simulink model "gm_ZynqBF_2tx_fpga"  (R2018b)
settings: Solver=FixedStepDiscrete  StartTime=0.0  StopTime=10.0  FixedStep=(1/420e3)/128  RelTol=1e-3
undefined symbols (not defined in the file or in its folder): a, b, c
libraries: hdlsllib x873, simulink x349
(part 37 of 40)

== system gm_ZynqBF_2tx_fpga/channel_estimator/peakdetect_ch2/correlator2/sum_elements_q_instance4 ==
  din : Inport  OutDataTypeStr=fixdt(1, 32, 16)  PortDimensions=[8]  SampleTime=1.86011904761905e-08
  start : Inport  Port=2  OutDataTypeStr=boolean  PortDimensions=1  SampleTime=1.86011904761905e-08
  Add : Sum  AccumDataTypeStr=fixdt(1, 33, 16)  OutDataTypeStr=fixdt(1, 32, 16)  SampleTime=1.86011904761905e-08
  Compare To Constant1 : simulink/Logic and Bit Operations/Compare To Constant  relop===  const=fi(0,0,3,0,'hex','7')  OutDataTypeStr=boolean
  Compare To Constant2 : simulink/Logic and Bit Operations/Compare To Constant  relop===  const=fi(0,0,1,0,'hex','1')  OutDataTypeStr=boolean
  Constant : Constant  Value=0  OutDataTypeStr=fixdt(1, 32, 16)  SampleTime=-1
  Constant1 : Constant  Value=0  OutDataTypeStr=fixdt(1, 16, 15)  SampleTime=-1
  Data Type Conversion : DataTypeConversion  OutDataTypeStr=uint8  SampleTime=1.86011904761905e-08
  Delay1 : Delay  DelayLength=double(1)  InitialCondition=0  InputProcessing=Inherited  SampleTime=1.86011904761905e-08
  HDL Counter : hdlsllib/Sources/HDL Counter  CountType=Free running  CountInit=double(0)  CountStep=double(1)  CountMax=25  CountFromType=Initial value  CountFrom=double(0)  CountResetPort=on  CountLoadPort=off  CountEnbPort=on  CountDirPort=off  CountDataType=Unsigned  CountWordLen=3  CountFracLen=0  CountSampTime=1.86011904761905e-08
      settings: SourceProductBaseCode=HD
  HDL Counter1 : hdlsllib/Sources/HDL Counter  CountType=Free running  CountInit=double(0)  CountStep=double(1)  CountMax=25  CountFromType=Initial value  CountFrom=double(0)  CountResetPort=off  CountLoadPort=off  CountEnbPort=on  CountDirPort=off  CountDataType=Unsigned  CountWordLen=1  CountFracLen=0  CountSampTime=1.86011904761905e-08
      settings: SourceProductBaseCode=HD
  Logical Operator : Logic  Operator=OR  AllPortsSameDT=off  OutDataTypeStr=boolean  SampleTime=1.86011904761905e-08
  Selector : Selector  IndexMode=Zero-based  SampleTime=1.86011904761905e-08  IndexOptions=Starting index (port)  Indices=double([1 3])  OutputSizes=double(1)
  Switch : Switch  Criteria=u2 ~= 0  Threshold=double(0)  OutDataTypeStr=fixdt(1, 32, 16)  SampleTime=1.86011904761905e-08
  Switch1 : Switch  Criteria=u2 ~= 0  Threshold=double(0)  OutDataTypeStr=fixdt(1, 32, 16)  SampleTime=1.86011904761905e-08
  dout : Outport
  vout : Outport  Port=2
  wires:
  Switch/1 -> Add/2
  Delay1/1 -> Switch/3
  HDL Counter1/1 -> Compare To Constant2/1
  Logical Operator/1 -> HDL Counter1/1
  start/1 -> Switch/2, HDL Counter/1, Logical Operator/1
  din/1 -> Selector/1
  Add/1 -> Delay1/1, dout/1
  Compare To Constant1/1 -> Logical Operator/2, vout/1
  Compare To Constant2/1 -> HDL Counter/2, Switch1/2
  Constant/1 -> Switch/1
  Constant1/1 -> Switch1/3
  Data Type Conversion/1 -> Selector/2
  HDL Counter/1 -> Compare To Constant1/1, Data Type Conversion/1
  Selector/1 -> Switch1/1
  Switch1/1 -> Add/1

== system gm_ZynqBF_2tx_fpga/channel_estimator/peakdetect_ch2/correlator2/sum_elements_q_instance5 ==
  din : Inport  OutDataTypeStr=fixdt(1, 32, 16)  PortDimensions=[8]  SampleTime=1.86011904761905e-08
  start : Inport  Port=2  OutDataTypeStr=boolean  PortDimensions=1  SampleTime=1.86011904761905e-08
  Add : Sum  AccumDataTypeStr=fixdt(1, 33, 16)  OutDataTypeStr=fixdt(1, 32, 16)  SampleTime=1.86011904761905e-08
  Compare To Constant1 : simulink/Logic and Bit Operations/Compare To Constant  relop===  const=fi(0,0,3,0,'hex','7')  OutDataTypeStr=boolean
  Compare To Constant2 : simulink/Logic and Bit Operations/Compare To Constant  relop===  const=fi(0,0,1,0,'hex','1')  OutDataTypeStr=boolean
  Constant : Constant  Value=0  OutDataTypeStr=fixdt(1, 32, 16)  SampleTime=-1
  Constant1 : Constant  Value=0  OutDataTypeStr=fixdt(1, 16, 15)  SampleTime=-1
  Data Type Conversion : DataTypeConversion  OutDataTypeStr=uint8  SampleTime=1.86011904761905e-08
  Delay1 : Delay  DelayLength=double(1)  InitialCondition=0  InputProcessing=Inherited  SampleTime=1.86011904761905e-08
  HDL Counter : hdlsllib/Sources/HDL Counter  CountType=Free running  CountInit=double(0)  CountStep=double(1)  CountMax=25  CountFromType=Initial value  CountFrom=double(0)  CountResetPort=on  CountLoadPort=off  CountEnbPort=on  CountDirPort=off  CountDataType=Unsigned  CountWordLen=3  CountFracLen=0  CountSampTime=1.86011904761905e-08
      settings: SourceProductBaseCode=HD
  HDL Counter1 : hdlsllib/Sources/HDL Counter  CountType=Free running  CountInit=double(0)  CountStep=double(1)  CountMax=25  CountFromType=Initial value  CountFrom=double(0)  CountResetPort=off  CountLoadPort=off  CountEnbPort=on  CountDirPort=off  CountDataType=Unsigned  CountWordLen=1  CountFracLen=0  CountSampTime=1.86011904761905e-08
      settings: SourceProductBaseCode=HD
  Logical Operator : Logic  Operator=OR  AllPortsSameDT=off  OutDataTypeStr=boolean  SampleTime=1.86011904761905e-08
  Selector : Selector  IndexMode=Zero-based  SampleTime=1.86011904761905e-08  IndexOptions=Starting index (port)  Indices=double([1 3])  OutputSizes=double(1)
  Switch : Switch  Criteria=u2 ~= 0  Threshold=double(0)  OutDataTypeStr=fixdt(1, 32, 16)  SampleTime=1.86011904761905e-08
  Switch1 : Switch  Criteria=u2 ~= 0  Threshold=double(0)  OutDataTypeStr=fixdt(1, 32, 16)  SampleTime=1.86011904761905e-08
  dout : Outport
  vout : Outport  Port=2
  wires:
  Switch/1 -> Add/2
  Delay1/1 -> Switch/3
  HDL Counter1/1 -> Compare To Constant2/1
  Logical Operator/1 -> HDL Counter1/1
  start/1 -> Switch/2, HDL Counter/1, Logical Operator/1
  din/1 -> Selector/1
  Add/1 -> Delay1/1, dout/1
  Compare To Constant1/1 -> Logical Operator/2, vout/1
  Compare To Constant2/1 -> HDL Counter/2, Switch1/2
  Constant/1 -> Switch/1
  Constant1/1 -> Switch1/3
  Data Type Conversion/1 -> Selector/2
  HDL Counter/1 -> Compare To Constant1/1, Data Type Conversion/1
  Selector/1 -> Switch1/1
  Switch1/1 -> Add/1

== system gm_ZynqBF_2tx_fpga/channel_estimator/peakdetect_ch2/correlator2/sum_elements_q_instance6 ==
  din : Inport  OutDataTypeStr=fixdt(1, 32, 16)  PortDimensions=[8]  SampleTime=1.86011904761905e-08
  start : Inport  Port=2  OutDataTypeStr=boolean  PortDimensions=1  SampleTime=1.86011904761905e-08
  Add : Sum  AccumDataTypeStr=fixdt(1, 33, 16)  OutDataTypeStr=fixdt(1, 32, 16)  SampleTime=1.86011904761905e-08
  Compare To Constant1 : simulink/Logic and Bit Operations/Compare To Constant  relop===  const=fi(0,0,3,0,'hex','7')  OutDataTypeStr=boolean
  Compare To Constant2 : simulink/Logic and Bit Operations/Compare To Constant  relop===  const=fi(0,0,1,0,'hex','1')  OutDataTypeStr=boolean
  Constant : Constant  Value=0  OutDataTypeStr=fixdt(1, 32, 16)  SampleTime=-1
  Constant1 : Constant  Value=0  OutDataTypeStr=fixdt(1, 16, 15)  SampleTime=-1
  Data Type Conversion : DataTypeConversion  OutDataTypeStr=uint8  SampleTime=1.86011904761905e-08
  Delay1 : Delay  DelayLength=double(1)  InitialCondition=0  InputProcessing=Inherited  SampleTime=1.86011904761905e-08
  HDL Counter : hdlsllib/Sources/HDL Counter  CountType=Free running  CountInit=double(0)  CountStep=double(1)  CountMax=25  CountFromType=Initial value  CountFrom=double(0)  CountResetPort=on  CountLoadPort=off  CountEnbPort=on  CountDirPort=off  CountDataType=Unsigned  CountWordLen=3  CountFracLen=0  CountSampTime=1.86011904761905e-08
      settings: SourceProductBaseCode=HD
  HDL Counter1 : hdlsllib/Sources/HDL Counter  CountType=Free running  CountInit=double(0)  CountStep=double(1)  CountMax=25  CountFromType=Initial value  CountFrom=double(0)  CountResetPort=off  CountLoadPort=off  CountEnbPort=on  CountDirPort=off  CountDataType=Unsigned  CountWordLen=1  CountFracLen=0  CountSampTime=1.86011904761905e-08
      settings: SourceProductBaseCode=HD
  Logical Operator : Logic  Operator=OR  AllPortsSameDT=off  OutDataTypeStr=boolean  SampleTime=1.86011904761905e-08
  Selector : Selector  IndexMode=Zero-based  SampleTime=1.86011904761905e-08  IndexOptions=Starting index (port)  Indices=double([1 3])  OutputSizes=double(1)
  Switch : Switch  Criteria=u2 ~= 0  Threshold=double(0)  OutDataTypeStr=fixdt(1, 32, 16)  SampleTime=1.86011904761905e-08
  Switch1 : Switch  Criteria=u2 ~= 0  Threshold=double(0)  OutDataTypeStr=fixdt(1, 32, 16)  SampleTime=1.86011904761905e-08
  dout : Outport
  vout : Outport  Port=2
  wires:
  Switch/1 -> Add/2
  Delay1/1 -> Switch/3
  HDL Counter1/1 -> Compare To Constant2/1
  Logical Operator/1 -> HDL Counter1/1
  start/1 -> Switch/2, HDL Counter/1, Logical Operator/1
  din/1 -> Selector/1
  Add/1 -> Delay1/1, dout/1
  Compare To Constant1/1 -> Logical Operator/2, vout/1
  Compare To Constant2/1 -> HDL Counter/2, Switch1/2
  Constant/1 -> Switch/1
  Constant1/1 -> Switch1/3
  Data Type Conversion/1 -> Selector/2
  HDL Counter/1 -> Compare To Constant1/1, Data Type Conversion/1
  Selector/1 -> Switch1/1
  Switch1/1 -> Add/1

== system gm_ZynqBF_2tx_fpga/channel_estimator/peakdetect_ch2/correlator2/sum_elements_q_instance7 ==
  din : Inport  OutDataTypeStr=fixdt(1, 32, 16)  PortDimensions=[8]  SampleTime=1.86011904761905e-08
  start : Inport  Port=2  OutDataTypeStr=boolean  PortDimensions=1  SampleTime=1.86011904761905e-08
  Add : Sum  AccumDataTypeStr=fixdt(1, 33, 16)  OutDataTypeStr=fixdt(1, 32, 16)  SampleTime=1.86011904761905e-08
  Compare To Constant1 : simulink/Logic and Bit Operations/Compare To Constant  relop===  const=fi(0,0,3,0,'hex','7')  OutDataTypeStr=boolean
  Compare To Constant2 : simulink/Logic and Bit Operations/Compare To Constant  relop===  const=fi(0,0,1,0,'hex','1')  OutDataTypeStr=boolean
  Constant : Constant  Value=0  OutDataTypeStr=fixdt(1, 32, 16)  SampleTime=-1
  Constant1 : Constant  Value=0  OutDataTypeStr=fixdt(1, 16, 15)  SampleTime=-1
  Data Type Conversion : DataTypeConversion  OutDataTypeStr=uint8  SampleTime=1.86011904761905e-08
  Delay1 : Delay  DelayLength=double(1)  InitialCondition=0  InputProcessing=Inherited  SampleTime=1.86011904761905e-08
  HDL Counter : hdlsllib/Sources/HDL Counter  CountType=Free running  CountInit=double(0)  CountStep=double(1)  CountMax=25  CountFromType=Initial value  CountFrom=double(0)  CountResetPort=on  CountLoadPort=off  CountEnbPort=on  CountDirPort=off  CountDataType=Unsigned  CountWordLen=3  CountFracLen=0  CountSampTime=1.86011904761905e-08
      settings: SourceProductBaseCode=HD
  HDL Counter1 : hdlsllib/Sources/HDL Counter  CountType=Free running  CountInit=double(0)  CountStep=double(1)  CountMax=25  CountFromType=Initial value  CountFrom=double(0)  CountResetPort=off  CountLoadPort=off  CountEnbPort=on  CountDirPort=off  CountDataType=Unsigned  CountWordLen=1  CountFracLen=0  CountSampTime=1.86011904761905e-08
      settings: SourceProductBaseCode=HD
  Logical Operator : Logic  Operator=OR  AllPortsSameDT=off  OutDataTypeStr=boolean  SampleTime=1.86011904761905e-08
  Selector : Selector  IndexMode=Zero-based  SampleTime=1.86011904761905e-08  IndexOptions=Starting index (port)  Indices=double([1 3])  OutputSizes=double(1)
  Switch : Switch  Criteria=u2 ~= 0  Threshold=double(0)  OutDataTypeStr=fixdt(1, 32, 16)  SampleTime=1.86011904761905e-08
  Switch1 : Switch  Criteria=u2 ~= 0  Threshold=double(0)  OutDataTypeStr=fixdt(1, 32, 16)  SampleTime=1.86011904761905e-08
  dout : Outport
  vout : Outport  Port=2
  wires:
  Switch/1 -> Add/2
  Delay1/1 -> Switch/3
  HDL Counter1/1 -> Compare To Constant2/1
  Logical Operator/1 -> HDL Counter1/1
  start/1 -> Switch/2, HDL Counter/1, Logical Operator/1
  din/1 -> Selector/1
  Add/1 -> Delay1/1, dout/1
  Compare To Constant1/1 -> Logical Operator/2, vout/1
  Compare To Constant2/1 -> HDL Counter/2, Switch1/2
  Constant/1 -> Switch/1
  Constant1/1 -> Switch1/3
  Data Type Conversion/1 -> Selector/2
  HDL Counter/1 -> Compare To Constant1/1, Data Type Conversion/1
  Selector/1 -> Switch1/1
  Switch1/1 -> Add/1

== system gm_ZynqBF_2tx_fpga/channel_estimator/peakdetect_ch2/correlator2/sum_elements_q_instance8 ==
  din : Inport  OutDataTypeStr=fixdt(1, 32, 16)  PortDimensions=[8]  SampleTime=1.86011904761905e-08
  start : Inport  Port=2  OutDataTypeStr=boolean  PortDimensions=1  SampleTime=1.86011904761905e-08
  Add : Sum  AccumDataTypeStr=fixdt(1, 33, 16)  OutDataTypeStr=fixdt(1, 32, 16)  SampleTime=1.86011904761905e-08
  Compare To Constant1 : simulink/Logic and Bit Operations/Compare To Constant  relop===  const=fi(0,0,3,0,'hex','7')  OutDataTypeStr=boolean
  Compare To Constant2 : simulink/Logic and Bit Operations/Compare To Constant  relop===  const=fi(0,0,1,0,'hex','1')  OutDataTypeStr=boolean
  Constant : Constant  Value=0  OutDataTypeStr=fixdt(1, 32, 16)  SampleTime=-1
  Constant1 : Constant  Value=0  OutDataTypeStr=fixdt(1, 16, 15)  SampleTime=-1
  Data Type Conversion : DataTypeConversion  OutDataTypeStr=uint8  SampleTime=1.86011904761905e-08
  Delay1 : Delay  DelayLength=double(1)  InitialCondition=0  InputProcessing=Inherited  SampleTime=1.86011904761905e-08
  HDL Counter : hdlsllib/Sources/HDL Counter  CountType=Free running  CountInit=double(0)  CountStep=double(1)  CountMax=25  CountFromType=Initial value  CountFrom=double(0)  CountResetPort=on  CountLoadPort=off  CountEnbPort=on  CountDirPort=off  CountDataType=Unsigned  CountWordLen=3  CountFracLen=0  CountSampTime=1.86011904761905e-08
      settings: SourceProductBaseCode=HD
  HDL Counter1 : hdlsllib/Sources/HDL Counter  CountType=Free running  CountInit=double(0)  CountStep=double(1)  CountMax=25  CountFromType=Initial value  CountFrom=double(0)  CountResetPort=off  CountLoadPort=off  CountEnbPort=on  CountDirPort=off  CountDataType=Unsigned  CountWordLen=1  CountFracLen=0  CountSampTime=1.86011904761905e-08
      settings: SourceProductBaseCode=HD
  Logical Operator : Logic  Operator=OR  AllPortsSameDT=off  OutDataTypeStr=boolean  SampleTime=1.86011904761905e-08
  Selector : Selector  IndexMode=Zero-based  SampleTime=1.86011904761905e-08  IndexOptions=Starting index (port)  Indices=double([1 3])  OutputSizes=double(1)
  Switch : Switch  Criteria=u2 ~= 0  Threshold=double(0)  OutDataTypeStr=fixdt(1, 32, 16)  SampleTime=1.86011904761905e-08
  Switch1 : Switch  Criteria=u2 ~= 0  Threshold=double(0)  OutDataTypeStr=fixdt(1, 32, 16)  SampleTime=1.86011904761905e-08
  dout : Outport
  vout : Outport  Port=2
  wires:
  Switch/1 -> Add/2
  Delay1/1 -> Switch/3
  HDL Counter1/1 -> Compare To Constant2/1
  Logical Operator/1 -> HDL Counter1/1
  start/1 -> Switch/2, HDL Counter/1, Logical Operator/1
  din/1 -> Selector/1
  Add/1 -> Delay1/1, dout/1
  Compare To Constant1/1 -> Logical Operator/2, vout/1
  Compare To Constant2/1 -> HDL Counter/2, Switch1/2
  Constant/1 -> Switch/1
  Constant1/1 -> Switch1/3
  Data Type Conversion/1 -> Selector/2
  HDL Counter/1 -> Compare To Constant1/1, Data Type Conversion/1
  Selector/1 -> Switch1/1
  Switch1/1 -> Add/1

== system gm_ZynqBF_2tx_fpga/channel_estimator/peakdetect_ch1/correlator1/rx_ram_i_instance1/get_bit ==
  u : Inport  OutDataTypeStr=fixdt(0, 64, 0)  PortDimensions=1  SampleTime=1.86011904761905e-08
  ind : Inport  Port=2  OutDataTypeStr=fixdt(0, 9, 0)  PortDimensions=1  SampleTime=1.86011904761905e-08
  get_bit : MATLAB Function  TreatAsAtomicUnit=on
  y : Outport
  wires:
  u/1 -> get_bit/1(u)
  ind/1 -> get_bit/2(ind)
  get_bit/1(y) -> y/1

== system gm_ZynqBF_2tx_fpga/channel_estimator/peakdetect_ch1/correlator1/rx_ram_i_instance10/get_bit ==
  u : Inport  OutDataTypeStr=fixdt(0, 64, 0)  PortDimensions=1  SampleTime=1.86011904761905e-08
  ind : Inport  Port=2  OutDataTypeStr=fixdt(0, 9, 0)  PortDimensions=1  SampleTime=1.86011904761905e-08
  get_bit : MATLAB Function  TreatAsAtomicUnit=on
  y : Outport
  wires:
  get_bit/1(y) -> y/1
  ind/1 -> get_bit/2(ind)
  u/1 -> get_bit/1(u)

== system gm_ZynqBF_2tx_fpga/channel_estimator/peakdetect_ch1/correlator1/rx_ram_i_instance11/get_bit ==
  u : Inport  OutDataTypeStr=fixdt(0, 64, 0)  PortDimensions=1  SampleTime=1.86011904761905e-08
  ind : Inport  Port=2  OutDataTypeStr=fixdt(0, 9, 0)  PortDimensions=1  SampleTime=1.86011904761905e-08
  get_bit : MATLAB Function  TreatAsAtomicUnit=on
  y : Outport
  wires:
  get_bit/1(y) -> y/1
  ind/1 -> get_bit/2(ind)
  u/1 -> get_bit/1(u)

== system gm_ZynqBF_2tx_fpga/channel_estimator/peakdetect_ch1/correlator1/rx_ram_i_instance12/get_bit ==
  u : Inport  OutDataTypeStr=fixdt(0, 64, 0)  PortDimensions=1  SampleTime=1.86011904761905e-08
  ind : Inport  Port=2  OutDataTypeStr=fixdt(0, 9, 0)  PortDimensions=1  SampleTime=1.86011904761905e-08
  get_bit : MATLAB Function  TreatAsAtomicUnit=on
  y : Outport
  wires:
  get_bit/1(y) -> y/1
  ind/1 -> get_bit/2(ind)
  u/1 -> get_bit/1(u)

== system gm_ZynqBF_2tx_fpga/channel_estimator/peakdetect_ch1/correlator1/rx_ram_i_instance13/get_bit ==
  u : Inport  OutDataTypeStr=fixdt(0, 64, 0)  PortDimensions=1  SampleTime=1.86011904761905e-08
  ind : Inport  Port=2  OutDataTypeStr=fixdt(0, 9, 0)  PortDimensions=1  SampleTime=1.86011904761905e-08
  get_bit : MATLAB Function  TreatAsAtomicUnit=on
  y : Outport
  wires:
  get_bit/1(y) -> y/1
  ind/1 -> get_bit/2(ind)
  u/1 -> get_bit/1(u)

== system gm_ZynqBF_2tx_fpga/channel_estimator/peakdetect_ch1/correlator1/rx_ram_i_instance14/get_bit ==
  u : Inport  OutDataTypeStr=fixdt(0, 64, 0)  PortDimensions=1  SampleTime=1.86011904761905e-08
  ind : Inport  Port=2  OutDataTypeStr=fixdt(0, 9, 0)  PortDimensions=1  SampleTime=1.86011904761905e-08
  get_bit : MATLAB Function  TreatAsAtomicUnit=on
  y : Outport
  wires:
  get_bit/1(y) -> y/1
  ind/1 -> get_bit/2(ind)
  u/1 -> get_bit/1(u)

== system gm_ZynqBF_2tx_fpga/channel_estimator/peakdetect_ch1/correlator1/rx_ram_i_instance15/get_bit ==
  u : Inport  OutDataTypeStr=fixdt(0, 64, 0)  PortDimensions=1  SampleTime=1.86011904761905e-08
  ind : Inport  Port=2  OutDataTypeStr=fixdt(0, 9, 0)  PortDimensions=1  SampleTime=1.86011904761905e-08
  get_bit : MATLAB Function  TreatAsAtomicUnit=on
  y : Outport
  wires:
  get_bit/1(y) -> y/1
  ind/1 -> get_bit/2(ind)
  u/1 -> get_bit/1(u)

== system gm_ZynqBF_2tx_fpga/channel_estimator/peakdetect_ch1/correlator1/rx_ram_i_instance16/get_bit ==
  u : Inport  OutDataTypeStr=fixdt(0, 64, 0)  PortDimensions=1  SampleTime=1.86011904761905e-08
  ind : Inport  Port=2  OutDataTypeStr=fixdt(0, 9, 0)  PortDimensions=1  SampleTime=1.86011904761905e-08
  get_bit : MATLAB Function  TreatAsAtomicUnit=on
  y : Outport
  wires:
  get_bit/1(y) -> y/1
  ind/1 -> get_bit/2(ind)
  u/1 -> get_bit/1(u)

== system gm_ZynqBF_2tx_fpga/channel_estimator/peakdetect_ch1/correlator1/rx_ram_i_instance17/get_bit ==
  u : Inport  OutDataTypeStr=fixdt(0, 64, 0)  PortDimensions=1  SampleTime=1.86011904761905e-08
  ind : Inport  Port=2  OutDataTypeStr=fixdt(0, 9, 0)  PortDimensions=1  SampleTime=1.86011904761905e-08
  get_bit : MATLAB Function  TreatAsAtomicUnit=on
  y : Outport
  wires:
  get_bit/1(y) -> y/1
  ind/1 -> get_bit/2(ind)
  u/1 -> get_bit/1(u)

== system gm_ZynqBF_2tx_fpga/channel_estimator/peakdetect_ch1/correlator1/rx_ram_i_instance18/get_bit ==
  u : Inport  OutDataTypeStr=fixdt(0, 64, 0)  PortDimensions=1  SampleTime=1.86011904761905e-08
  ind : Inport  Port=2  OutDataTypeStr=fixdt(0, 9, 0)  PortDimensions=1  SampleTime=1.86011904761905e-08
  get_bit : MATLAB Function  TreatAsAtomicUnit=on
  y : Outport
  wires:
  get_bit/1(y) -> y/1
  ind/1 -> get_bit/2(ind)
  u/1 -> get_bit/1(u)

== system gm_ZynqBF_2tx_fpga/channel_estimator/peakdetect_ch1/correlator1/rx_ram_i_instance19/get_bit ==
  u : Inport  OutDataTypeStr=fixdt(0, 64, 0)  PortDimensions=1  SampleTime=1.86011904761905e-08
  ind : Inport  Port=2  OutDataTypeStr=fixdt(0, 9, 0)  PortDimensions=1  SampleTime=1.86011904761905e-08
  get_bit : MATLAB Function  TreatAsAtomicUnit=on
  y : Outport
  wires:
  get_bit/1(y) -> y/1
  ind/1 -> get_bit/2(ind)
  u/1 -> get_bit/1(u)

== system gm_ZynqBF_2tx_fpga/channel_estimator/peakdetect_ch1/correlator1/rx_ram_i_instance2/get_bit ==
  u : Inport  OutDataTypeStr=fixdt(0, 64, 0)  PortDimensions=1  SampleTime=1.86011904761905e-08
  ind : Inport  Port=2  OutDataTypeStr=fixdt(0, 9, 0)  PortDimensions=1  SampleTime=1.86011904761905e-08
  get_bit : MATLAB Function  TreatAsAtomicUnit=on
  y : Outport
  wires:
  get_bit/1(y) -> y/1
  ind/1 -> get_bit/2(ind)
  u/1 -> get_bit/1(u)

== system gm_ZynqBF_2tx_fpga/channel_estimator/peakdetect_ch1/correlator1/rx_ram_i_instance20/get_bit ==
  u : Inport  OutDataTypeStr=fixdt(0, 64, 0)  PortDimensions=1  SampleTime=1.86011904761905e-08
  ind : Inport  Port=2  OutDataTypeStr=fixdt(0, 9, 0)  PortDimensions=1  SampleTime=1.86011904761905e-08
  get_bit : MATLAB Function  TreatAsAtomicUnit=on
  y : Outport
  wires:
  get_bit/1(y) -> y/1
  ind/1 -> get_bit/2(ind)
  u/1 -> get_bit/1(u)

== system gm_ZynqBF_2tx_fpga/channel_estimator/peakdetect_ch1/correlator1/rx_ram_i_instance21/get_bit ==
  u : Inport  OutDataTypeStr=fixdt(0, 64, 0)  PortDimensions=1  SampleTime=1.86011904761905e-08
  ind : Inport  Port=2  OutDataTypeStr=fixdt(0, 9, 0)  PortDimensions=1  SampleTime=1.86011904761905e-08
  get_bit : MATLAB Function  TreatAsAtomicUnit=on
  y : Outport
  wires:
  get_bit/1(y) -> y/1
  ind/1 -> get_bit/2(ind)
  u/1 -> get_bit/1(u)

== system gm_ZynqBF_2tx_fpga/channel_estimator/peakdetect_ch1/correlator1/rx_ram_i_instance22/get_bit ==
  u : Inport  OutDataTypeStr=fixdt(0, 64, 0)  PortDimensions=1  SampleTime=1.86011904761905e-08
  ind : Inport  Port=2  OutDataTypeStr=fixdt(0, 9, 0)  PortDimensions=1  SampleTime=1.86011904761905e-08
  get_bit : MATLAB Function  TreatAsAtomicUnit=on
  y : Outport
  wires:
  get_bit/1(y) -> y/1
  ind/1 -> get_bit/2(ind)
  u/1 -> get_bit/1(u)

== system gm_ZynqBF_2tx_fpga/channel_estimator/peakdetect_ch1/correlator1/rx_ram_i_instance23/get_bit ==
  u : Inport  OutDataTypeStr=fixdt(0, 64, 0)  PortDimensions=1  SampleTime=1.86011904761905e-08
  ind : Inport  Port=2  OutDataTypeStr=fixdt(0, 9, 0)  PortDimensions=1  SampleTime=1.86011904761905e-08
  get_bit : MATLAB Function  TreatAsAtomicUnit=on
  y : Outport
  wires:
  get_bit/1(y) -> y/1
  ind/1 -> get_bit/2(ind)
  u/1 -> get_bit/1(u)

== system gm_ZynqBF_2tx_fpga/channel_estimator/peakdetect_ch1/correlator1/rx_ram_i_instance24/get_bit ==
  u : Inport  OutDataTypeStr=fixdt(0, 64, 0)  PortDimensions=1  SampleTime=1.86011904761905e-08
  ind : Inport  Port=2  OutDataTypeStr=fixdt(0, 9, 0)  PortDimensions=1  SampleTime=1.86011904761905e-08
  get_bit : MATLAB Function  TreatAsAtomicUnit=on
  y : Outport
  wires:
  get_bit/1(y) -> y/1
  ind/1 -> get_bit/2(ind)
  u/1 -> get_bit/1(u)

== system gm_ZynqBF_2tx_fpga/channel_estimator/peakdetect_ch1/correlator1/rx_ram_i_instance25/get_bit ==
  u : Inport  OutDataTypeStr=fixdt(0, 64, 0)  PortDimensions=1  SampleTime=1.86011904761905e-08
  ind : Inport  Port=2  OutDataTypeStr=fixdt(0, 9, 0)  PortDimensions=1  SampleTime=1.86011904761905e-08
  get_bit : MATLAB Function  TreatAsAtomicUnit=on
  y : Outport
  wires:
  get_bit/1(y) -> y/1
  ind/1 -> get_bit/2(ind)
  u/1 -> get_bit/1(u)

== system gm_ZynqBF_2tx_fpga/channel_estimator/peakdetect_ch1/correlator1/rx_ram_i_instance26/get_bit ==
  u : Inport  OutDataTypeStr=fixdt(0, 64, 0)  PortDimensions=1  SampleTime=1.86011904761905e-08
  ind : Inport  Port=2  OutDataTypeStr=fixdt(0, 9, 0)  PortDimensions=1  SampleTime=1.86011904761905e-08
  get_bit : MATLAB Function  TreatAsAtomicUnit=on
  y : Outport
  wires:
  get_bit/1(y) -> y/1
  ind/1 -> get_bit/2(ind)
  u/1 -> get_bit/1(u)

== system gm_ZynqBF_2tx_fpga/channel_estimator/peakdetect_ch1/correlator1/rx_ram_i_instance27/get_bit ==
  u : Inport  OutDataTypeStr=fixdt(0, 64, 0)  PortDimensions=1  SampleTime=1.86011904761905e-08
  ind : Inport  Port=2  OutDataTypeStr=fixdt(0, 9, 0)  PortDimensions=1  SampleTime=1.86011904761905e-08
  get_bit : MATLAB Function  TreatAsAtomicUnit=on
  y : Outport
  wires:
  get_bit/1(y) -> y/1
  ind/1 -> get_bit/2(ind)
  u/1 -> get_bit/1(u)

== system gm_ZynqBF_2tx_fpga/channel_estimator/peakdetect_ch1/correlator1/rx_ram_i_instance28/get_bit ==
  u : Inport  OutDataTypeStr=fixdt(0, 64, 0)  PortDimensions=1  SampleTime=1.86011904761905e-08
  ind : Inport  Port=2  OutDataTypeStr=fixdt(0, 9, 0)  PortDimensions=1  SampleTime=1.86011904761905e-08
  get_bit : MATLAB Function  TreatAsAtomicUnit=on
  y : Outport
  wires:
  get_bit/1(y) -> y/1
  ind/1 -> get_bit/2(ind)
  u/1 -> get_bit/1(u)

== system gm_ZynqBF_2tx_fpga/channel_estimator/peakdetect_ch1/correlator1/rx_ram_i_instance29/get_bit ==
  u : Inport  OutDataTypeStr=fixdt(0, 64, 0)  PortDimensions=1  SampleTime=1.86011904761905e-08
  ind : Inport  Port=2  OutDataTypeStr=fixdt(0, 9, 0)  PortDimensions=1  SampleTime=1.86011904761905e-08
  get_bit : MATLAB Function  TreatAsAtomicUnit=on
  y : Outport
  wires:
  get_bit/1(y) -> y/1
  ind/1 -> get_bit/2(ind)
  u/1 -> get_bit/1(u)

== system gm_ZynqBF_2tx_fpga/channel_estimator/peakdetect_ch1/correlator1/rx_ram_i_instance3/get_bit ==
  u : Inport  OutDataTypeStr=fixdt(0, 64, 0)  PortDimensions=1  SampleTime=1.86011904761905e-08
  ind : Inport  Port=2  OutDataTypeStr=fixdt(0, 9, 0)  PortDimensions=1  SampleTime=1.86011904761905e-08
  get_bit : MATLAB Function  TreatAsAtomicUnit=on
  y : Outport
  wires:
  get_bit/1(y) -> y/1
  ind/1 -> get_bit/2(ind)
  u/1 -> get_bit/1(u)

== system gm_ZynqBF_2tx_fpga/channel_estimator/peakdetect_ch1/correlator1/rx_ram_i_instance30/get_bit ==
  u : Inport  OutDataTypeStr=fixdt(0, 64, 0)  PortDimensions=1  SampleTime=1.86011904761905e-08
  ind : Inport  Port=2  OutDataTypeStr=fixdt(0, 9, 0)  PortDimensions=1  SampleTime=1.86011904761905e-08
  get_bit : MATLAB Function  TreatAsAtomicUnit=on
  y : Outport
  wires:
  get_bit/1(y) -> y/1
  ind/1 -> get_bit/2(ind)
  u/1 -> get_bit/1(u)

== system gm_ZynqBF_2tx_fpga/channel_estimator/peakdetect_ch1/correlator1/rx_ram_i_instance31/get_bit ==
  u : Inport  OutDataTypeStr=fixdt(0, 64, 0)  PortDimensions=1  SampleTime=1.86011904761905e-08
  ind : Inport  Port=2  OutDataTypeStr=fixdt(0, 9, 0)  PortDimensions=1  SampleTime=1.86011904761905e-08
  get_bit : MATLAB Function  TreatAsAtomicUnit=on
  y : Outport
  wires:
  get_bit/1(y) -> y/1
  ind/1 -> get_bit/2(ind)
  u/1 -> get_bit/1(u)

== system gm_ZynqBF_2tx_fpga/channel_estimator/peakdetect_ch1/correlator1/rx_ram_i_instance32/get_bit ==
  u : Inport  OutDataTypeStr=fixdt(0, 64, 0)  PortDimensions=1  SampleTime=1.86011904761905e-08
  ind : Inport  Port=2  OutDataTypeStr=fixdt(0, 9, 0)  PortDimensions=1  SampleTime=1.86011904761905e-08
  get_bit : MATLAB Function  TreatAsAtomicUnit=on
  y : Outport
  wires:
  get_bit/1(y) -> y/1
  ind/1 -> get_bit/2(ind)
  u/1 -> get_bit/1(u)

== system gm_ZynqBF_2tx_fpga/channel_estimator/peakdetect_ch1/correlator1/rx_ram_i_instance33/get_bit ==
  u : Inport  OutDataTypeStr=fixdt(0, 64, 0)  PortDimensions=1  SampleTime=1.86011904761905e-08
  ind : Inport  Port=2  OutDataTypeStr=fixdt(0, 9, 0)  PortDimensions=1  SampleTime=1.86011904761905e-08
  get_bit : MATLAB Function  TreatAsAtomicUnit=on
  y : Outport
  wires:
  get_bit/1(y) -> y/1
  ind/1 -> get_bit/2(ind)
  u/1 -> get_bit/1(u)

== system gm_ZynqBF_2tx_fpga/channel_estimator/peakdetect_ch1/correlator1/rx_ram_i_instance34/get_bit ==
  u : Inport  OutDataTypeStr=fixdt(0, 64, 0)  PortDimensions=1  SampleTime=1.86011904761905e-08
  ind : Inport  Port=2  OutDataTypeStr=fixdt(0, 9, 0)  PortDimensions=1  SampleTime=1.86011904761905e-08
  get_bit : MATLAB Function  TreatAsAtomicUnit=on
  y : Outport
  wires:
  get_bit/1(y) -> y/1
  ind/1 -> get_bit/2(ind)
  u/1 -> get_bit/1(u)

== system gm_ZynqBF_2tx_fpga/channel_estimator/peakdetect_ch1/correlator1/rx_ram_i_instance35/get_bit ==
  u : Inport  OutDataTypeStr=fixdt(0, 64, 0)  PortDimensions=1  SampleTime=1.86011904761905e-08
  ind : Inport  Port=2  OutDataTypeStr=fixdt(0, 9, 0)  PortDimensions=1  SampleTime=1.86011904761905e-08
  get_bit : MATLAB Function  TreatAsAtomicUnit=on
  y : Outport
  wires:
  get_bit/1(y) -> y/1
  ind/1 -> get_bit/2(ind)
  u/1 -> get_bit/1(u)

== system gm_ZynqBF_2tx_fpga/channel_estimator/peakdetect_ch1/correlator1/rx_ram_i_instance36/get_bit ==
  u : Inport  OutDataTypeStr=fixdt(0, 64, 0)  PortDimensions=1  SampleTime=1.86011904761905e-08
  ind : Inport  Port=2  OutDataTypeStr=fixdt(0, 9, 0)  PortDimensions=1  SampleTime=1.86011904761905e-08
  get_bit : MATLAB Function  TreatAsAtomicUnit=on
  y : Outport
  wires:
  get_bit/1(y) -> y/1
  ind/1 -> get_bit/2(ind)
  u/1 -> get_bit/1(u)

== system gm_ZynqBF_2tx_fpga/channel_estimator/peakdetect_ch1/correlator1/rx_ram_i_instance37/get_bit ==
  u : Inport  OutDataTypeStr=fixdt(0, 64, 0)  PortDimensions=1  SampleTime=1.86011904761905e-08
  ind : Inport  Port=2  OutDataTypeStr=fixdt(0, 9, 0)  PortDimensions=1  SampleTime=1.86011904761905e-08
  get_bit : MATLAB Function  TreatAsAtomicUnit=on
  y : Outport
  wires:
  get_bit/1(y) -> y/1
  ind/1 -> get_bit/2(ind)
  u/1 -> get_bit/1(u)

== system gm_ZynqBF_2tx_fpga/channel_estimator/peakdetect_ch1/correlator1/rx_ram_i_instance38/get_bit ==
  u : Inport  OutDataTypeStr=fixdt(0, 64, 0)  PortDimensions=1  SampleTime=1.86011904761905e-08
  ind : Inport  Port=2  OutDataTypeStr=fixdt(0, 9, 0)  PortDimensions=1  SampleTime=1.86011904761905e-08
  get_bit : MATLAB Function  TreatAsAtomicUnit=on
  y : Outport
  wires:
  get_bit/1(y) -> y/1
  ind/1 -> get_bit/2(ind)
  u/1 -> get_bit/1(u)

== system gm_ZynqBF_2tx_fpga/channel_estimator/peakdetect_ch1/correlator1/rx_ram_i_instance39/get_bit ==
  u : Inport  OutDataTypeStr=fixdt(0, 64, 0)  PortDimensions=1  SampleTime=1.86011904761905e-08
  ind : Inport  Port=2  OutDataTypeStr=fixdt(0, 9, 0)  PortDimensions=1  SampleTime=1.86011904761905e-08
  get_bit : MATLAB Function  TreatAsAtomicUnit=on
  y : Outport
  wires:
  get_bit/1(y) -> y/1
  ind/1 -> get_bit/2(ind)
  u/1 -> get_bit/1(u)

== system gm_ZynqBF_2tx_fpga/channel_estimator/peakdetect_ch1/correlator1/rx_ram_i_instance4/get_bit ==
  u : Inport  OutDataTypeStr=fixdt(0, 64, 0)  PortDimensions=1  SampleTime=1.86011904761905e-08
  ind : Inport  Port=2  OutDataTypeStr=fixdt(0, 9, 0)  PortDimensions=1  SampleTime=1.86011904761905e-08
  get_bit : MATLAB Function  TreatAsAtomicUnit=on
  y : Outport
  wires:
  get_bit/1(y) -> y/1
  ind/1 -> get_bit/2(ind)
  u/1 -> get_bit/1(u)

== system gm_ZynqBF_2tx_fpga/channel_estimator/peakdetect_ch1/correlator1/rx_ram_i_instance40/get_bit ==
  u : Inport  OutDataTypeStr=fixdt(0, 64, 0)  PortDimensions=1  SampleTime=1.86011904761905e-08
  ind : Inport  Port=2  OutDataTypeStr=fixdt(0, 9, 0)  PortDimensions=1  SampleTime=1.86011904761905e-08
  get_bit : MATLAB Function  TreatAsAtomicUnit=on
  y : Outport
  wires:
  get_bit/1(y) -> y/1
  ind/1 -> get_bit/2(ind)
  u/1 -> get_bit/1(u)

== system gm_ZynqBF_2tx_fpga/channel_estimator/peakdetect_ch1/correlator1/rx_ram_i_instance41/get_bit ==
  u : Inport  OutDataTypeStr=fixdt(0, 64, 0)  PortDimensions=1  SampleTime=1.86011904761905e-08
  ind : Inport  Port=2  OutDataTypeStr=fixdt(0, 9, 0)  PortDimensions=1  SampleTime=1.86011904761905e-08
  get_bit : MATLAB Function  TreatAsAtomicUnit=on
  y : Outport
  wires:
  get_bit/1(y) -> y/1
  ind/1 -> get_bit/2(ind)
  u/1 -> get_bit/1(u)

== system gm_ZynqBF_2tx_fpga/channel_estimator/peakdetect_ch1/correlator1/rx_ram_i_instance42/get_bit ==
  u : Inport  OutDataTypeStr=fixdt(0, 64, 0)  PortDimensions=1  SampleTime=1.86011904761905e-08
  ind : Inport  Port=2  OutDataTypeStr=fixdt(0, 9, 0)  PortDimensions=1  SampleTime=1.86011904761905e-08
  get_bit : MATLAB Function  TreatAsAtomicUnit=on
  y : Outport
  wires:
  get_bit/1(y) -> y/1
  ind/1 -> get_bit/2(ind)
  u/1 -> get_bit/1(u)

== system gm_ZynqBF_2tx_fpga/channel_estimator/peakdetect_ch1/correlator1/rx_ram_i_instance43/get_bit ==
  u : Inport  OutDataTypeStr=fixdt(0, 64, 0)  PortDimensions=1  SampleTime=1.86011904761905e-08
  ind : Inport  Port=2  OutDataTypeStr=fixdt(0, 9, 0)  PortDimensions=1  SampleTime=1.86011904761905e-08
  get_bit : MATLAB Function  TreatAsAtomicUnit=on
  y : Outport
  wires:
  get_bit/1(y) -> y/1
  ind/1 -> get_bit/2(ind)
  u/1 -> get_bit/1(u)

== system gm_ZynqBF_2tx_fpga/channel_estimator/peakdetect_ch1/correlator1/rx_ram_i_instance44/get_bit ==
  u : Inport  OutDataTypeStr=fixdt(0, 64, 0)  PortDimensions=1  SampleTime=1.86011904761905e-08
  ind : Inport  Port=2  OutDataTypeStr=fixdt(0, 9, 0)  PortDimensions=1  SampleTime=1.86011904761905e-08
  get_bit : MATLAB Function  TreatAsAtomicUnit=on
  y : Outport
  wires:
  get_bit/1(y) -> y/1
  ind/1 -> get_bit/2(ind)
  u/1 -> get_bit/1(u)

== system gm_ZynqBF_2tx_fpga/channel_estimator/peakdetect_ch1/correlator1/rx_ram_i_instance45/get_bit ==
  u : Inport  OutDataTypeStr=fixdt(0, 64, 0)  PortDimensions=1  SampleTime=1.86011904761905e-08
  ind : Inport  Port=2  OutDataTypeStr=fixdt(0, 9, 0)  PortDimensions=1  SampleTime=1.86011904761905e-08
  get_bit : MATLAB Function  TreatAsAtomicUnit=on
  y : Outport
  wires:
  get_bit/1(y) -> y/1
  ind/1 -> get_bit/2(ind)
  u/1 -> get_bit/1(u)

== system gm_ZynqBF_2tx_fpga/channel_estimator/peakdetect_ch1/correlator1/rx_ram_i_instance46/get_bit ==
  u : Inport  OutDataTypeStr=fixdt(0, 64, 0)  PortDimensions=1  SampleTime=1.86011904761905e-08
  ind : Inport  Port=2  OutDataTypeStr=fixdt(0, 9, 0)  PortDimensions=1  SampleTime=1.86011904761905e-08
  get_bit : MATLAB Function  TreatAsAtomicUnit=on
  y : Outport
  wires:
  get_bit/1(y) -> y/1
  ind/1 -> get_bit/2(ind)
  u/1 -> get_bit/1(u)

== system gm_ZynqBF_2tx_fpga/channel_estimator/peakdetect_ch1/correlator1/rx_ram_i_instance47/get_bit ==
  u : Inport  OutDataTypeStr=fixdt(0, 64, 0)  PortDimensions=1  SampleTime=1.86011904761905e-08
  ind : Inport  Port=2  OutDataTypeStr=fixdt(0, 9, 0)  PortDimensions=1  SampleTime=1.86011904761905e-08
  get_bit : MATLAB Function  TreatAsAtomicUnit=on
  y : Outport
  wires:
  get_bit/1(y) -> y/1
  ind/1 -> get_bit/2(ind)
  u/1 -> get_bit/1(u)

== system gm_ZynqBF_2tx_fpga/channel_estimator/peakdetect_ch1/correlator1/rx_ram_i_instance48/get_bit ==
  u : Inport  OutDataTypeStr=fixdt(0, 64, 0)  PortDimensions=1  SampleTime=1.86011904761905e-08
  ind : Inport  Port=2  OutDataTypeStr=fixdt(0, 9, 0)  PortDimensions=1  SampleTime=1.86011904761905e-08
  get_bit : MATLAB Function  TreatAsAtomicUnit=on
  y : Outport
  wires:
  get_bit/1(y) -> y/1
  ind/1 -> get_bit/2(ind)
  u/1 -> get_bit/1(u)

== system gm_ZynqBF_2tx_fpga/channel_estimator/peakdetect_ch1/correlator1/rx_ram_i_instance49/get_bit ==
  u : Inport  OutDataTypeStr=fixdt(0, 64, 0)  PortDimensions=1  SampleTime=1.86011904761905e-08
  ind : Inport  Port=2  OutDataTypeStr=fixdt(0, 9, 0)  PortDimensions=1  SampleTime=1.86011904761905e-08
  get_bit : MATLAB Function  TreatAsAtomicUnit=on
  y : Outport
  wires:
  get_bit/1(y) -> y/1
  ind/1 -> get_bit/2(ind)
  u/1 -> get_bit/1(u)

== system gm_ZynqBF_2tx_fpga/channel_estimator/peakdetect_ch1/correlator1/rx_ram_i_instance5/get_bit ==
  u : Inport  OutDataTypeStr=fixdt(0, 64, 0)  PortDimensions=1  SampleTime=1.86011904761905e-08
  ind : Inport  Port=2  OutDataTypeStr=fixdt(0, 9, 0)  PortDimensions=1  SampleTime=1.86011904761905e-08
  get_bit : MATLAB Function  TreatAsAtomicUnit=on
  y : Outport
  wires:
  get_bit/1(y) -> y/1
  ind/1 -> get_bit/2(ind)
  u/1 -> get_bit/1(u)

== system gm_ZynqBF_2tx_fpga/channel_estimator/peakdetect_ch1/correlator1/rx_ram_i_instance50/get_bit ==
  u : Inport  OutDataTypeStr=fixdt(0, 64, 0)  PortDimensions=1  SampleTime=1.86011904761905e-08
  ind : Inport  Port=2  OutDataTypeStr=fixdt(0, 9, 0)  PortDimensions=1  SampleTime=1.86011904761905e-08
  get_bit : MATLAB Function  TreatAsAtomicUnit=on
  y : Outport
  wires:
  get_bit/1(y) -> y/1
  ind/1 -> get_bit/2(ind)
  u/1 -> get_bit/1(u)

== system gm_ZynqBF_2tx_fpga/channel_estimator/peakdetect_ch1/correlator1/rx_ram_i_instance51/get_bit ==
  u : Inport  OutDataTypeStr=fixdt(0, 64, 0)  PortDimensions=1  SampleTime=1.86011904761905e-08
  ind : Inport  Port=2  OutDataTypeStr=fixdt(0, 9, 0)  PortDimensions=1  SampleTime=1.86011904761905e-08
  get_bit : MATLAB Function  TreatAsAtomicUnit=on
  y : Outport
  wires:
  get_bit/1(y) -> y/1
  ind/1 -> get_bit/2(ind)
  u/1 -> get_bit/1(u)

== system gm_ZynqBF_2tx_fpga/channel_estimator/peakdetect_ch1/correlator1/rx_ram_i_instance52/get_bit ==
  u : Inport  OutDataTypeStr=fixdt(0, 64, 0)  PortDimensions=1  SampleTime=1.86011904761905e-08
  ind : Inport  Port=2  OutDataTypeStr=fixdt(0, 9, 0)  PortDimensions=1  SampleTime=1.86011904761905e-08
  get_bit : MATLAB Function  TreatAsAtomicUnit=on
  y : Outport
  wires:
  get_bit/1(y) -> y/1
  ind/1 -> get_bit/2(ind)
  u/1 -> get_bit/1(u)

== system gm_ZynqBF_2tx_fpga/channel_estimator/peakdetect_ch1/correlator1/rx_ram_i_instance53/get_bit ==
  u : Inport  OutDataTypeStr=fixdt(0, 64, 0)  PortDimensions=1  SampleTime=1.86011904761905e-08
  ind : Inport  Port=2  OutDataTypeStr=fixdt(0, 9, 0)  PortDimensions=1  SampleTime=1.86011904761905e-08
  get_bit : MATLAB Function  TreatAsAtomicUnit=on
  y : Outport
  wires:
  get_bit/1(y) -> y/1
  ind/1 -> get_bit/2(ind)
  u/1 -> get_bit/1(u)

== system gm_ZynqBF_2tx_fpga/channel_estimator/peakdetect_ch1/correlator1/rx_ram_i_instance54/get_bit ==
  u : Inport  OutDataTypeStr=fixdt(0, 64, 0)  PortDimensions=1  SampleTime=1.86011904761905e-08
  ind : Inport  Port=2  OutDataTypeStr=fixdt(0, 9, 0)  PortDimensions=1  SampleTime=1.86011904761905e-08
  get_bit : MATLAB Function  TreatAsAtomicUnit=on
  y : Outport
  wires:
  get_bit/1(y) -> y/1
  ind/1 -> get_bit/2(ind)
  u/1 -> get_bit/1(u)

== system gm_ZynqBF_2tx_fpga/channel_estimator/peakdetect_ch1/correlator1/rx_ram_i_instance55/get_bit ==
  u : Inport  OutDataTypeStr=fixdt(0, 64, 0)  PortDimensions=1  SampleTime=1.86011904761905e-08
  ind : Inport  Port=2  OutDataTypeStr=fixdt(0, 9, 0)  PortDimensions=1  SampleTime=1.86011904761905e-08
  get_bit : MATLAB Function  TreatAsAtomicUnit=on
  y : Outport
  wires:
  get_bit/1(y) -> y/1
  ind/1 -> get_bit/2(ind)
  u/1 -> get_bit/1(u)

== system gm_ZynqBF_2tx_fpga/channel_estimator/peakdetect_ch1/correlator1/rx_ram_i_instance56/get_bit ==
  u : Inport  OutDataTypeStr=fixdt(0, 64, 0)  PortDimensions=1  SampleTime=1.86011904761905e-08
  ind : Inport  Port=2  OutDataTypeStr=fixdt(0, 9, 0)  PortDimensions=1  SampleTime=1.86011904761905e-08
  get_bit : MATLAB Function  TreatAsAtomicUnit=on
  y : Outport
  wires:
  get_bit/1(y) -> y/1
  ind/1 -> get_bit/2(ind)
  u/1 -> get_bit/1(u)

== system gm_ZynqBF_2tx_fpga/channel_estimator/peakdetect_ch1/correlator1/rx_ram_i_instance57/get_bit ==
  u : Inport  OutDataTypeStr=fixdt(0, 64, 0)  PortDimensions=1  SampleTime=1.86011904761905e-08
  ind : Inport  Port=2  OutDataTypeStr=fixdt(0, 9, 0)  PortDimensions=1  SampleTime=1.86011904761905e-08
  get_bit : MATLAB Function  TreatAsAtomicUnit=on
  y : Outport
  wires:
  get_bit/1(y) -> y/1
  ind/1 -> get_bit/2(ind)
  u/1 -> get_bit/1(u)

== system gm_ZynqBF_2tx_fpga/channel_estimator/peakdetect_ch1/correlator1/rx_ram_i_instance58/get_bit ==
  u : Inport  OutDataTypeStr=fixdt(0, 64, 0)  PortDimensions=1  SampleTime=1.86011904761905e-08
  ind : Inport  Port=2  OutDataTypeStr=fixdt(0, 9, 0)  PortDimensions=1  SampleTime=1.86011904761905e-08
  get_bit : MATLAB Function  TreatAsAtomicUnit=on
  y : Outport
  wires:
  get_bit/1(y) -> y/1
  ind/1 -> get_bit/2(ind)
  u/1 -> get_bit/1(u)

== system gm_ZynqBF_2tx_fpga/channel_estimator/peakdetect_ch1/correlator1/rx_ram_i_instance59/get_bit ==
  u : Inport  OutDataTypeStr=fixdt(0, 64, 0)  PortDimensions=1  SampleTime=1.86011904761905e-08
  ind : Inport  Port=2  OutDataTypeStr=fixdt(0, 9, 0)  PortDimensions=1  SampleTime=1.86011904761905e-08
  get_bit : MATLAB Function  TreatAsAtomicUnit=on
  y : Outport
  wires:
  get_bit/1(y) -> y/1
  ind/1 -> get_bit/2(ind)
  u/1 -> get_bit/1(u)

== system gm_ZynqBF_2tx_fpga/channel_estimator/peakdetect_ch1/correlator1/rx_ram_i_instance6/get_bit ==
  u : Inport  OutDataTypeStr=fixdt(0, 64, 0)  PortDimensions=1  SampleTime=1.86011904761905e-08
  ind : Inport  Port=2  OutDataTypeStr=fixdt(0, 9, 0)  PortDimensions=1  SampleTime=1.86011904761905e-08
  get_bit : MATLAB Function  TreatAsAtomicUnit=on
  y : Outport
  wires:
  get_bit/1(y) -> y/1
  ind/1 -> get_bit/2(ind)
  u/1 -> get_bit/1(u)

== system gm_ZynqBF_2tx_fpga/channel_estimator/peakdetect_ch1/correlator1/rx_ram_i_instance60/get_bit ==
  u : Inport  OutDataTypeStr=fixdt(0, 64, 0)  PortDimensions=1  SampleTime=1.86011904761905e-08
  ind : Inport  Port=2  OutDataTypeStr=fixdt(0, 9, 0)  PortDimensions=1  SampleTime=1.86011904761905e-08
  get_bit : MATLAB Function  TreatAsAtomicUnit=on
  y : Outport
  wires:
  get_bit/1(y) -> y/1
  ind/1 -> get_bit/2(ind)
  u/1 -> get_bit/1(u)

== system gm_ZynqBF_2tx_fpga/channel_estimator/peakdetect_ch1/correlator1/rx_ram_i_instance61/get_bit ==
  u : Inport  OutDataTypeStr=fixdt(0, 64, 0)  PortDimensions=1  SampleTime=1.86011904761905e-08
  ind : Inport  Port=2  OutDataTypeStr=fixdt(0, 9, 0)  PortDimensions=1  SampleTime=1.86011904761905e-08
  get_bit : MATLAB Function  TreatAsAtomicUnit=on
  y : Outport
  wires:
  get_bit/1(y) -> y/1
  ind/1 -> get_bit/2(ind)
  u/1 -> get_bit/1(u)

== system gm_ZynqBF_2tx_fpga/channel_estimator/peakdetect_ch1/correlator1/rx_ram_i_instance62/get_bit ==
  u : Inport  OutDataTypeStr=fixdt(0, 64, 0)  PortDimensions=1  SampleTime=1.86011904761905e-08
  ind : Inport  Port=2  OutDataTypeStr=fixdt(0, 9, 0)  PortDimensions=1  SampleTime=1.86011904761905e-08
  get_bit : MATLAB Function  TreatAsAtomicUnit=on
  y : Outport
  wires:
  get_bit/1(y) -> y/1
  ind/1 -> get_bit/2(ind)
  u/1 -> get_bit/1(u)

== system gm_ZynqBF_2tx_fpga/channel_estimator/peakdetect_ch1/correlator1/rx_ram_i_instance63/get_bit ==
  u : Inport  OutDataTypeStr=fixdt(0, 64, 0)  PortDimensions=1  SampleTime=1.86011904761905e-08
  ind : Inport  Port=2  OutDataTypeStr=fixdt(0, 9, 0)  PortDimensions=1  SampleTime=1.86011904761905e-08
  get_bit : MATLAB Function  TreatAsAtomicUnit=on
  y : Outport
  wires:
  get_bit/1(y) -> y/1
  ind/1 -> get_bit/2(ind)
  u/1 -> get_bit/1(u)

== system gm_ZynqBF_2tx_fpga/channel_estimator/peakdetect_ch1/correlator1/rx_ram_i_instance64/get_bit ==
  u : Inport  OutDataTypeStr=fixdt(0, 64, 0)  PortDimensions=1  SampleTime=1.86011904761905e-08
  ind : Inport  Port=2  OutDataTypeStr=fixdt(0, 9, 0)  PortDimensions=1  SampleTime=1.86011904761905e-08
  get_bit : MATLAB Function  TreatAsAtomicUnit=on
  y : Outport
  wires:
  get_bit/1(y) -> y/1
  ind/1 -> get_bit/2(ind)
  u/1 -> get_bit/1(u)

== system gm_ZynqBF_2tx_fpga/channel_estimator/peakdetect_ch1/correlator1/rx_ram_i_instance7/get_bit ==
  u : Inport  OutDataTypeStr=fixdt(0, 64, 0)  PortDimensions=1  SampleTime=1.86011904761905e-08
  ind : Inport  Port=2  OutDataTypeStr=fixdt(0, 9, 0)  PortDimensions=1  SampleTime=1.86011904761905e-08
  get_bit : MATLAB Function  TreatAsAtomicUnit=on
  y : Outport
  wires:
  get_bit/1(y) -> y/1
  ind/1 -> get_bit/2(ind)
  u/1 -> get_bit/1(u)

== system gm_ZynqBF_2tx_fpga/channel_estimator/peakdetect_ch1/correlator1/rx_ram_i_instance8/get_bit ==
  u : Inport  OutDataTypeStr=fixdt(0, 64, 0)  PortDimensions=1  SampleTime=1.86011904761905e-08
  ind : Inport  Port=2  OutDataTypeStr=fixdt(0, 9, 0)  PortDimensions=1  SampleTime=1.86011904761905e-08
  get_bit : MATLAB Function  TreatAsAtomicUnit=on
  y : Outport
  wires:
  get_bit/1(y) -> y/1
  ind/1 -> get_bit/2(ind)
  u/1 -> get_bit/1(u)

== system gm_ZynqBF_2tx_fpga/channel_estimator/peakdetect_ch1/correlator1/rx_ram_i_instance9/get_bit ==
  u : Inport  OutDataTypeStr=fixdt(0, 64, 0)  PortDimensions=1  SampleTime=1.86011904761905e-08
  ind : Inport  Port=2  OutDataTypeStr=fixdt(0, 9, 0)  PortDimensions=1  SampleTime=1.86011904761905e-08
  get_bit : MATLAB Function  TreatAsAtomicUnit=on
  y : Outport
  wires:
  get_bit/1(y) -> y/1
  ind/1 -> get_bit/2(ind)
  u/1 -> get_bit/1(u)

== system gm_ZynqBF_2tx_fpga/channel_estimator/peakdetect_ch1/correlator1/rx_ram_q_instance1/get_bit ==
  u : Inport  OutDataTypeStr=fixdt(0, 64, 0)  PortDimensions=1  SampleTime=1.86011904761905e-08
  ind : Inport  Port=2  OutDataTypeStr=fixdt(0, 9, 0)  PortDimensions=1  SampleTime=1.86011904761905e-08
  get_bit : MATLAB Function  TreatAsAtomicUnit=on
  y : Outport
  wires:
  get_bit/1(y) -> y/1
  ind/1 -> get_bit/2(ind)
  u/1 -> get_bit/1(u)

== system gm_ZynqBF_2tx_fpga/channel_estimator/peakdetect_ch1/correlator1/rx_ram_q_instance10/get_bit ==
  u : Inport  OutDataTypeStr=fixdt(0, 64, 0)  PortDimensions=1  SampleTime=1.86011904761905e-08
  ind : Inport  Port=2  OutDataTypeStr=fixdt(0, 9, 0)  PortDimensions=1  SampleTime=1.86011904761905e-08
  get_bit : MATLAB Function  TreatAsAtomicUnit=on
  y : Outport
  wires:
  get_bit/1(y) -> y/1
  ind/1 -> get_bit/2(ind)
  u/1 -> get_bit/1(u)

== system gm_ZynqBF_2tx_fpga/channel_estimator/peakdetect_ch1/correlator1/rx_ram_q_instance11/get_bit ==
  u : Inport  OutDataTypeStr=fixdt(0, 64, 0)  PortDimensions=1  SampleTime=1.86011904761905e-08
  ind : Inport  Port=2  OutDataTypeStr=fixdt(0, 9, 0)  PortDimensions=1  SampleTime=1.86011904761905e-08
  get_bit : MATLAB Function  TreatAsAtomicUnit=on
  y : Outport
  wires:
  get_bit/1(y) -> y/1
  ind/1 -> get_bit/2(ind)
  u/1 -> get_bit/1(u)

== system gm_ZynqBF_2tx_fpga/channel_estimator/peakdetect_ch1/correlator1/rx_ram_q_instance12/get_bit ==
  u : Inport  OutDataTypeStr=fixdt(0, 64, 0)  PortDimensions=1  SampleTime=1.86011904761905e-08
  ind : Inport  Port=2  OutDataTypeStr=fixdt(0, 9, 0)  PortDimensions=1  SampleTime=1.86011904761905e-08
  get_bit : MATLAB Function  TreatAsAtomicUnit=on
  y : Outport
  wires:
  get_bit/1(y) -> y/1
  ind/1 -> get_bit/2(ind)
  u/1 -> get_bit/1(u)

== system gm_ZynqBF_2tx_fpga/channel_estimator/peakdetect_ch1/correlator1/rx_ram_q_instance13/get_bit ==
  u : Inport  OutDataTypeStr=fixdt(0, 64, 0)  PortDimensions=1  SampleTime=1.86011904761905e-08
  ind : Inport  Port=2  OutDataTypeStr=fixdt(0, 9, 0)  PortDimensions=1  SampleTime=1.86011904761905e-08
  get_bit : MATLAB Function  TreatAsAtomicUnit=on
  y : Outport
  wires:
  get_bit/1(y) -> y/1
  ind/1 -> get_bit/2(ind)
  u/1 -> get_bit/1(u)

== system gm_ZynqBF_2tx_fpga/channel_estimator/peakdetect_ch1/correlator1/rx_ram_q_instance14/get_bit ==
  u : Inport  OutDataTypeStr=fixdt(0, 64, 0)  PortDimensions=1  SampleTime=1.86011904761905e-08
  ind : Inport  Port=2  OutDataTypeStr=fixdt(0, 9, 0)  PortDimensions=1  SampleTime=1.86011904761905e-08
  get_bit : MATLAB Function  TreatAsAtomicUnit=on
  y : Outport
  wires:
  get_bit/1(y) -> y/1
  ind/1 -> get_bit/2(ind)
  u/1 -> get_bit/1(u)

== system gm_ZynqBF_2tx_fpga/channel_estimator/peakdetect_ch1/correlator1/rx_ram_q_instance15/get_bit ==
  u : Inport  OutDataTypeStr=fixdt(0, 64, 0)  PortDimensions=1  SampleTime=1.86011904761905e-08
  ind : Inport  Port=2  OutDataTypeStr=fixdt(0, 9, 0)  PortDimensions=1  SampleTime=1.86011904761905e-08
  get_bit : MATLAB Function  TreatAsAtomicUnit=on
  y : Outport
  wires:
  get_bit/1(y) -> y/1
  ind/1 -> get_bit/2(ind)
  u/1 -> get_bit/1(u)

== system gm_ZynqBF_2tx_fpga/channel_estimator/peakdetect_ch1/correlator1/rx_ram_q_instance16/get_bit ==
  u : Inport  OutDataTypeStr=fixdt(0, 64, 0)  PortDimensions=1  SampleTime=1.86011904761905e-08
  ind : Inport  Port=2  OutDataTypeStr=fixdt(0, 9, 0)  PortDimensions=1  SampleTime=1.86011904761905e-08
  get_bit : MATLAB Function  TreatAsAtomicUnit=on
  y : Outport
  wires:
  get_bit/1(y) -> y/1
  ind/1 -> get_bit/2(ind)
  u/1 -> get_bit/1(u)

== system gm_ZynqBF_2tx_fpga/channel_estimator/peakdetect_ch1/correlator1/rx_ram_q_instance17/get_bit ==
  u : Inport  OutDataTypeStr=fixdt(0, 64, 0)  PortDimensions=1  SampleTime=1.86011904761905e-08
  ind : Inport  Port=2  OutDataTypeStr=fixdt(0, 9, 0)  PortDimensions=1  SampleTime=1.86011904761905e-08
  get_bit : MATLAB Function  TreatAsAtomicUnit=on
  y : Outport
  wires:
  get_bit/1(y) -> y/1
  ind/1 -> get_bit/2(ind)
  u/1 -> get_bit/1(u)

== system gm_ZynqBF_2tx_fpga/channel_estimator/peakdetect_ch1/correlator1/rx_ram_q_instance18/get_bit ==
  u : Inport  OutDataTypeStr=fixdt(0, 64, 0)  PortDimensions=1  SampleTime=1.86011904761905e-08
  ind : Inport  Port=2  OutDataTypeStr=fixdt(0, 9, 0)  PortDimensions=1  SampleTime=1.86011904761905e-08
  get_bit : MATLAB Function  TreatAsAtomicUnit=on
  y : Outport
  wires:
  get_bit/1(y) -> y/1
  ind/1 -> get_bit/2(ind)
  u/1 -> get_bit/1(u)

== system gm_ZynqBF_2tx_fpga/channel_estimator/peakdetect_ch1/correlator1/rx_ram_q_instance19/get_bit ==
  u : Inport  OutDataTypeStr=fixdt(0, 64, 0)  PortDimensions=1  SampleTime=1.86011904761905e-08
  ind : Inport  Port=2  OutDataTypeStr=fixdt(0, 9, 0)  PortDimensions=1  SampleTime=1.86011904761905e-08
  get_bit : MATLAB Function  TreatAsAtomicUnit=on
  y : Outport
  wires:
  get_bit/1(y) -> y/1
  ind/1 -> get_bit/2(ind)
  u/1 -> get_bit/1(u)

== system gm_ZynqBF_2tx_fpga/channel_estimator/peakdetect_ch1/correlator1/rx_ram_q_instance2/get_bit ==
  u : Inport  OutDataTypeStr=fixdt(0, 64, 0)  PortDimensions=1  SampleTime=1.86011904761905e-08
  ind : Inport  Port=2  OutDataTypeStr=fixdt(0, 9, 0)  PortDimensions=1  SampleTime=1.86011904761905e-08
  get_bit : MATLAB Function  TreatAsAtomicUnit=on
  y : Outport
  wires:
  get_bit/1(y) -> y/1
  ind/1 -> get_bit/2(ind)
  u/1 -> get_bit/1(u)

== system gm_ZynqBF_2tx_fpga/channel_estimator/peakdetect_ch1/correlator1/rx_ram_q_instance20/get_bit ==
  u : Inport  OutDataTypeStr=fixdt(0, 64, 0)  PortDimensions=1  SampleTime=1.86011904761905e-08
  ind : Inport  Port=2  OutDataTypeStr=fixdt(0, 9, 0)  PortDimensions=1  SampleTime=1.86011904761905e-08
  get_bit : MATLAB Function  TreatAsAtomicUnit=on
  y : Outport
  wires:
  get_bit/1(y) -> y/1
  ind/1 -> get_bit/2(ind)
  u/1 -> get_bit/1(u)
